simulink model "LQR_obsv_sim"  (R2024b)
settings: Solver=ode5  StartTime=0.0  StopTime=10.0  FixedStep=0.001  RelTol=1e-3
undefined symbols (not defined in the file): A, B, C, K, L, x0, x_star
settings Model: Creator=johnc  LastModifiedBy=johnc

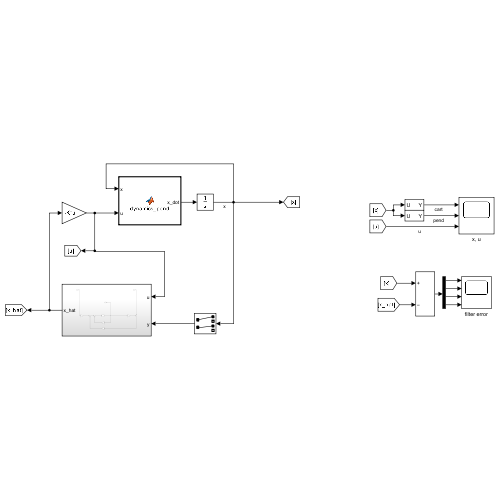
[thumbnail: Simulink's stored preview of the top-level diagram]
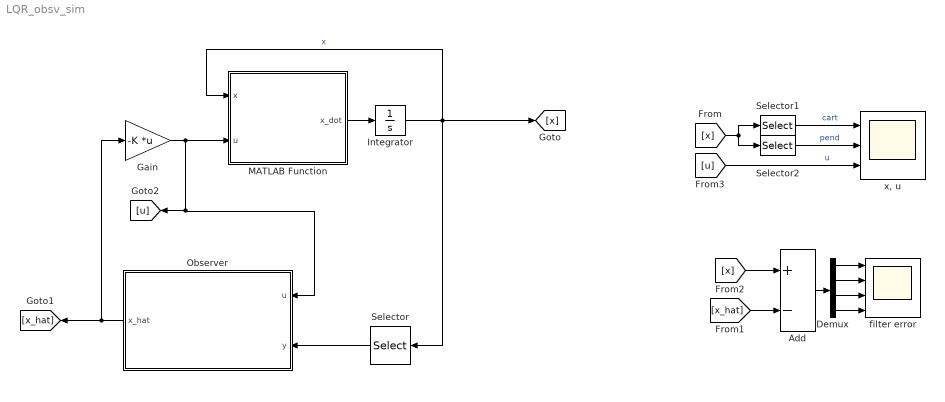
== system LQR_obsv_sim ==
  Add : Sum  Inputs=+-
  Demux : Demux
  Gain : Gain  Gain=-K  Multiplication=Matrix(K*u)
  Integrator : Integrator  InitialCondition=x0
  MATLAB Function : MATLAB Function  TreatAsAtomicUnit=on
  Observer : Subsystem
  Selector : Selector  InputPortWidth=4  IndexOptions=Index vector (dialog)  Indices=[1 3]  OutputSizes=1
  Selector1 : Selector  InputPortWidth=4  IndexOptions=Index vector (dialog)  Indices=[1 2]  OutputSizes=1
  Selector2 : Selector  InputPortWidth=4  IndexOptions=Index vector (dialog)  Indices=[3 4]  OutputSizes=1
  filter error : Scope  NumInputPorts=4
  "x, u" : Scope  NumInputPorts=3
  wires:
  MATLAB Function/1(x_dot) -> Integrator/1
  Integrator/1 -> Selector/1, [x], MATLAB Function/1(x)  "x"
  Selector/1 -> Observer/2(y)
  Observer/1(x_hat) -> Gain/1, [x_hat]
  Gain/1 -> Observer/1(u), [u], MATLAB Function/2(u)
  [x] -> Selector1/1, Selector2/1
  Selector1/1 -> "x, u"/1  "cart"
  Selector2/1 -> "x, u"/2  "pend"
  [x] -> Add/1
  [x_hat] -> Add/2
  Add/1 -> Demux/1
  Demux/1 -> filter error/1
  Demux/2 -> filter error/2
  Demux/3 -> filter error/3
  Demux/4 -> filter error/4
  [u] -> "x, u"/3  "u"

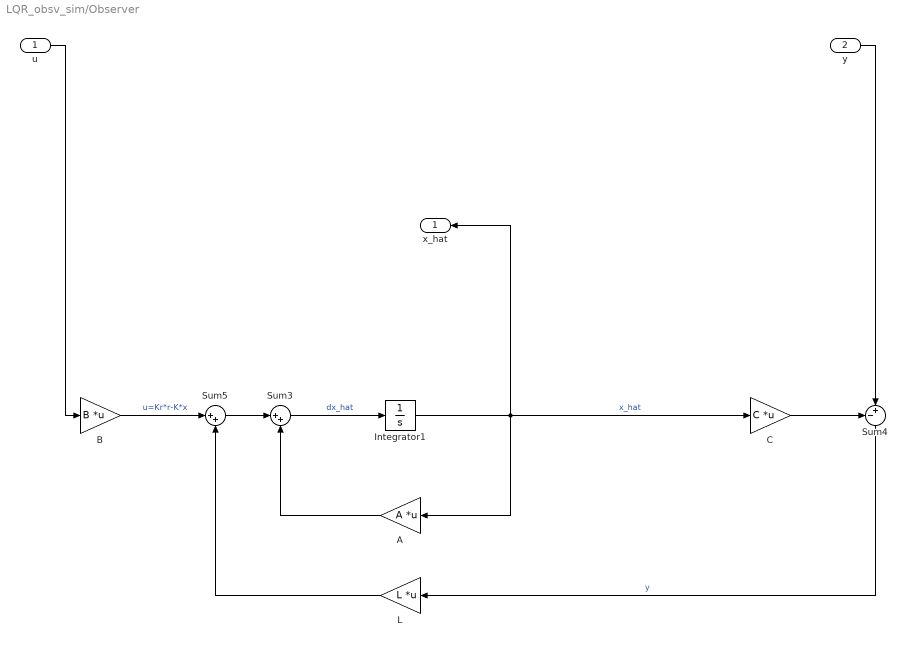
== system LQR_obsv_sim/Observer ==
  u : Inport
  y : Inport  Port=2
  A : Gain  Gain=A  Multiplication=Matrix(K*u)
  B : Gain  Gain=B  Multiplication=Matrix(K*u)
  C : Gain  Gain=C  Multiplication=Matrix(K*u)
  Integrator1 : Integrator  InitialCondition=x0-x_star
  L : Gain  Gain=L  Multiplication=Matrix(K*u)
  Sum3 : Sum  Inputs=|++
  Sum4 : Sum  Inputs=-+|
  Sum5 : Sum  Inputs=|++
  x_hat : Outport
  wires:
  C/1 -> Sum4/1
  Integrator1/1 -> x_hat/1, C/1, A/1  "x_hat"
  Sum5/1 -> Sum3/1
  L/1 -> Sum5/2
  A/1 -> Sum3/2
  Sum4/1 -> L/1  "y"
  Sum3/1 -> Integrator1/1  "dx_hat"
  B/1 -> Sum5/1  "u=Kr*r-K*x"
  u/1 -> B/1
  y/1 -> Sum4/2

== matlab function LQR_obsv_sim/MATLAB Function ==
  data: x input; x_dot output; u input; params parameter
function x_dot  = dynamics_pend(x, u, params)

g = params.g;
mc = params.mc;
mp = params.mp;
Jp = params.Jp;
bc = params.bc;
bp = params.bp;
Lp = params.Lp;
r_pulley = params.r_pulley;
Ke = params.Ke;

x1 = x(1);
x2 = x(2);
x3 = x(3);
x4 = x(4);

x1_dot = x2;
x2_dot = (Ke*u/r_pulley - bc*x2 - mp*Lp*x4^2*sin(x3) + mp*Lp*cos(x3)*(-bp*x4 + mp*g*Lp*sin(x3))/(mp*Lp^2 + Jp))*1/(mc + mp - mp^2*Lp^2*cos(x3)^2/(mp*Lp^2 + Jp));
x3_dot = x4;
x4_dot = (-bp*x4 + mp*g*Lp*sin(x3) + mp*Lp*cos(x3)*(Ke*u/r_pulley - bc*x2 - mp*Lp*x4^2*sin(x3))/(mc + mp))*1/(mp*Lp^2 + Jp - mp^2*Lp^2*cos(x3)^2/(mc + mp));

x_dot = [x1_dot; x2_dot; x3_dot; x4_dot];
